simulink model "MMC_idealarm_NLM_SwitchingModel_20251014"  (R2024b)
settings: Solver=FixedStepAuto  StartTime=t_init_sim  StopTime=sim_time  FixedStep=Ts  RelTol=1e-3
InitFcn:
  | param_armsim_20251013
StartFcn:
  | param_armsim_20251013
values from neighbouring files (symbols this model uses):
  a = 1    [param_armsim_20251013.m]
  C_m = 188.4e-6    (= 0.0001884)    [param_armsim_20251013.m]
  f0 = 500    [param_armsim_20251013.m]
  f_control = 10e3    (= 10000)    [param_armsim_20251013.m]
  Fc = 2.5e3    (= 2500)    [param_armsim_20251013.m]
  isAlgoTriActive = true    [param_armsim_20251013.m]
  isPWMActive = false    [param_armsim_20251013.m]
  L_ac = 30e-3    (= 0.03)    [param_armsim_20251013.m]
  m = 1    [param_armsim_20251013.m]
  N = 5    [param_armsim_20251013.m]
  phi = pi/2    (= 1.57079632679)    [param_armsim_20251013.m]
  R_ac = 6    [param_armsim_20251013.m]
  time_charge = 0.2    [param_armsim_20251013.m]
  Ts = 1e-6    (= 1e-06)    [param_armsim_20251013.m]
  VDC = 150    [param_armsim_20251013.m]
undefined symbols (not defined in the file or in its folder): C_SM
libraries: spsVoltageMeasurementLib x8, spsHalfBridgeMMCLib x5, spsSeriesRLCBranchLib x1, spsControlledVoltageSourceLib x1, spsCurrentMeasurementLib x1, spsDiodeLib x1, spsGroundLib x1, spsPWMGeneratorMultilevelLib x1, spspowerguiLib x1
settings Model: Creator=ana  LastModifiedBy=ana

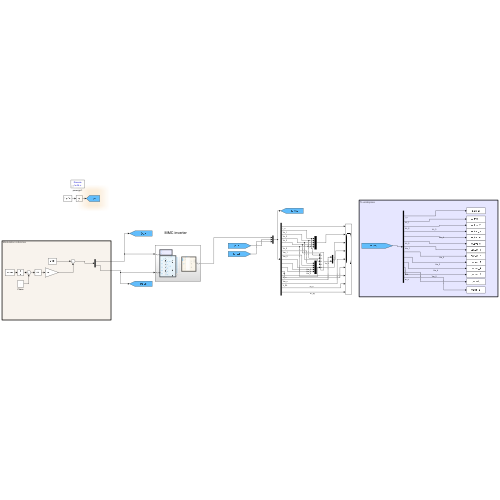
[thumbnail: Simulink's stored preview of the top-level diagram]
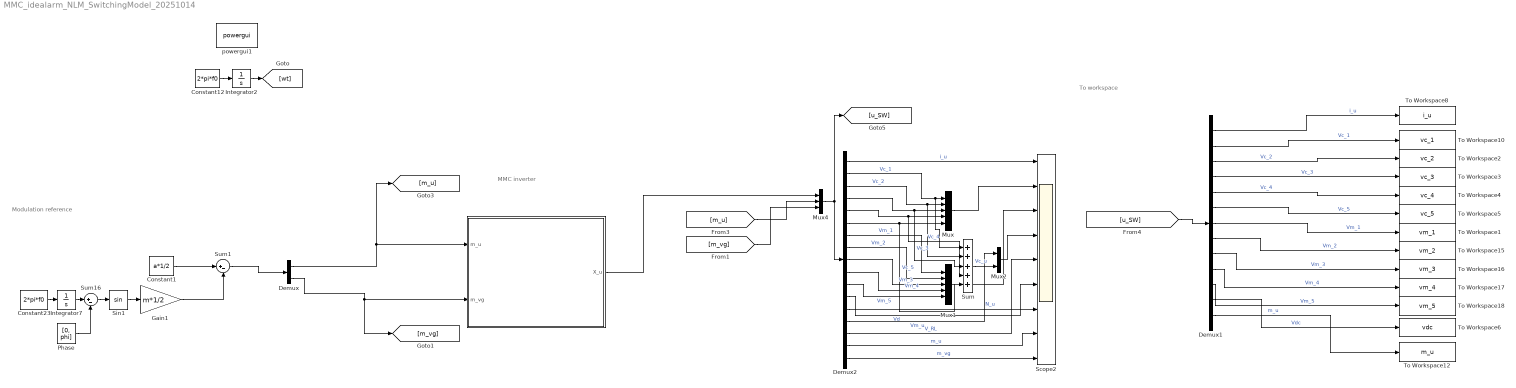
== system MMC_idealarm_NLM_SwitchingModel_20251014 ==
  note: MMC inverter
  note: To workspace
  note: Modulation reference
  " " : Subsystem
  Constant1 : Constant  Value=a*1/2
  Constant12 : Constant  Value=2*pi*f0
  Constant23 : Constant  Value=2*pi*f0
  Demux : Demux  Outputs=2
  Demux1 : Demux  Outputs=13
  Demux2 : Demux  Outputs=17
  Gain1 : Gain  Gain=m*1/2
  Integrator2 : Integrator
  Integrator7 : Integrator
  Mux : Mux  Inputs=5
  Mux1 : Mux  Inputs=5
  Mux2 : Mux  Inputs=2
  Mux4 : Mux  Inputs=3
  Phase : Constant  Value=[0, phi]
  Scope2 : Scope  NumInputPorts=9
  Sin1 : Trigonometry
  Sum : Sum  Inputs=+++++
  Sum1 : Sum  Inputs=|+-
  Sum16 : Sum  Inputs=|+-
  To Workspace1 : ToWorkspace  VariableName=vm_1  SaveFormat=Structure With Time  SampleTime=-1
      settings: MaxDataPoints=10*200000
  To Workspace10 : ToWorkspace  VariableName=vc_1  SaveFormat=Structure With Time  SampleTime=-1
      settings: MaxDataPoints=10*200000
  To Workspace12 : ToWorkspace  VariableName=m_u  SaveFormat=Structure With Time  SampleTime=-1
      settings: MaxDataPoints=10*200000
  To Workspace15 : ToWorkspace  VariableName=vm_2  SaveFormat=Structure With Time  SampleTime=-1
      settings: MaxDataPoints=10*200000
  To Workspace16 : ToWorkspace  VariableName=vm_3  SaveFormat=Structure With Time  SampleTime=-1
      settings: MaxDataPoints=10*200000
  To Workspace17 : ToWorkspace  VariableName=vm_4  SaveFormat=Structure With Time  SampleTime=-1
      settings: MaxDataPoints=10*200000
  To Workspace18 : ToWorkspace  VariableName=vm_5  SaveFormat=Structure With Time  SampleTime=-1
      settings: MaxDataPoints=10*200000
  To Workspace2 : ToWorkspace  VariableName=vc_2  SaveFormat=Structure With Time  SampleTime=-1
      settings: MaxDataPoints=10*200000
  To Workspace3 : ToWorkspace  VariableName=vc_3  SaveFormat=Structure With Time  SampleTime=-1
      settings: MaxDataPoints=10*200000
  To Workspace4 : ToWorkspace  VariableName=vc_4  SaveFormat=Structure With Time  SampleTime=-1
      settings: MaxDataPoints=10*200000
  To Workspace5 : ToWorkspace  VariableName=vc_5  SaveFormat=Structure With Time  SampleTime=-1
      settings: MaxDataPoints=10*200000
  To Workspace6 : ToWorkspace  VariableName=vdc  SaveFormat=Structure With Time  SampleTime=-1
      settings: MaxDataPoints=10*200000
  To Workspace8 : ToWorkspace  VariableName=i_u  SaveFormat=Structure With Time  SampleTime=-1
      settings: MaxDataPoints=10*200000
  powergui1 : spspowerguiLib/powergui  Priority=1  SimulationMode=Discrete  SampleTime=Ts  frequency=60  Iterations=50  frequencyindice=0  Pbase=100e6  ErrMax=1e-4  UnitsV=V  UnitsW=W  buscounter=0  FunctionMessages=off  echomessages=off  EnableUseOfTLC=off  CurrentSourceSwitches=off  DisableSnubberDevices=off  DisableRonSwitches=off  DisableVfSwitches=off  DisplayEquations=off  AutomaticDiscreteSolvers=off  SolverType=Backward Euler  Interpol=off  ExternalGateDelay=off  methode=off  Ts=0  x0status=blocks  SPID=off  SwTol=0  HookPort=off  NonlinearTolerance=1e-4  nMaxIteration=100  ContinueOnMaxIteration=off  RestoreLinks=warning  ResistiveCurrentMeasurement=off  Frange=[0:2:500]  Ylog=off  Xlog=on  ShowGrid=off  save=off  variable=ZData  structure=0  ZoomFFT=off  StartTime=0.0  cycles=1  DisplayStyle=1  fundamental=60  FreqAxis=off  MaxFrequency=1000  frequencyindicesteady=1  RmsSteady=1  display=off
  wires:
  Demux2/7 -> Mux1/1  "Vm_1"
  Demux2/11 -> Mux1/5  "Vm_5"
  Demux2/9 -> Mux1/3  "Vm_3"
  [u_SW] -> Demux1/1
  Demux1/8 -> To Workspace15/1  "Vm_2"
  Demux1/13 -> To Workspace12/1  "m_u"
  Demux2/10 -> Mux1/4  "Vm_4"
  Demux1/10 -> To Workspace17/1  "Vm_4"
  Demux1/5 -> To Workspace4/1  "Vc_4"
  Demux1/12 -> To Workspace6/1  "Vdc"
  Sin1/1 -> Gain1/1
  " "/1(X_u) -> Mux4/1
  Demux2/1 -> Scope2/1  "i_u"
  Sum16/1 -> Sin1/1
  Constant1/1 -> Sum1/1
  Constant23/1 -> Integrator7/1
  Demux2/16 -> Scope2/8  "m_u"
  Demux1/11 -> To Workspace18/1  "Vm_5"
  [m_u] -> Mux4/2
  Integrator7/1 -> Sum16/1
  Demux2/6 -> Sum/5, Mux/5  "Vc_5"
  Mux4/1 -> [u_SW], Demux2/1
  Constant12/1 -> Integrator2/1
  Integrator2/1 -> [wt]
  Demux1/9 -> To Workspace16/1  "Vm_3"
  Demux1/7 -> To Workspace1/1  "Vm_1"
  Demux1/3 -> To Workspace2/1  "Vc_2"
  Demux1/4 -> To Workspace3/1  "Vc_3"
  Demux1/6 -> To Workspace5/1  "Vc_5"
  Gain1/1 -> Sum1/2
  Phase/1 -> Sum16/2
  Demux1/2 -> To Workspace10/1  "Vc_1"
  Demux2/2 -> Sum/1, Mux/1  "Vc_1"
  Demux1/1 -> To Workspace8/1  "i_u"
  Demux2/5 -> Sum/4, Mux/4  "Vc_4"
  Demux2/3 -> Mux/2, Sum/2  "Vc_2"
  Demux2/4 -> Mux/3, Sum/3  "Vc_3"
  Mux/1 -> Scope2/2
  Demux2/8 -> Mux1/2  "Vm_2"
  Mux1/1 -> Scope2/3
  Demux2/13 -> Scope2/7  "N_u"
  Demux/1 -> [m_u], " "/1(m_u)
  Sum1/1 -> Demux/1
  Demux/2 -> " "/2(m_vg), [m_vg]
  [m_vg] -> Mux4/3
  Demux2/17 -> Scope2/9  "m_vg"
  Demux2/12 -> Scope2/6  "Vd"
  Demux2/15 -> Scope2/5  "V_RL"
  Sum/1 -> Mux2/2  "Vc_u"
  Mux2/1 -> Scope2/4
  Demux2/14 -> Mux2/1  "Vm_u"

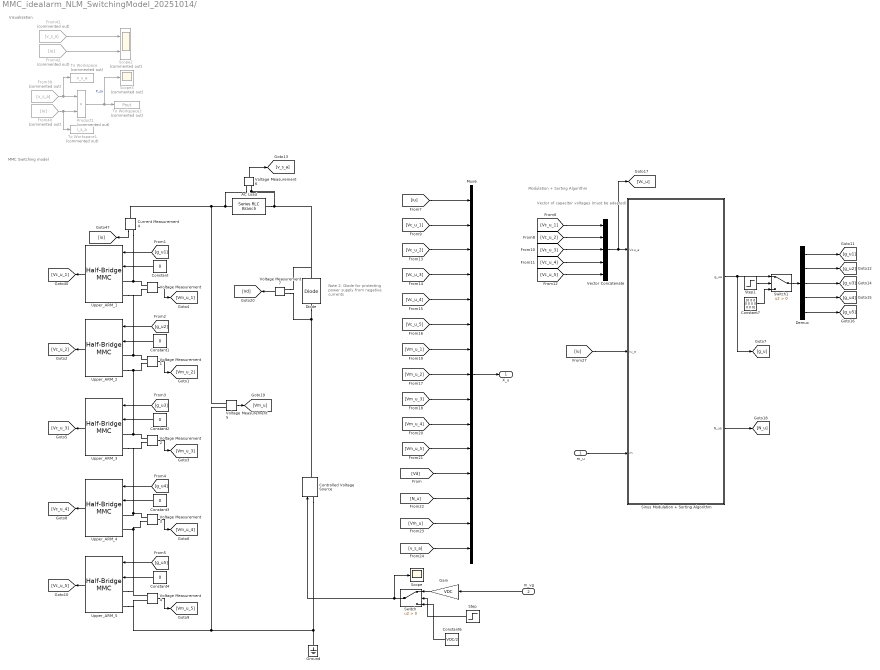
== system MMC_idealarm_NLM_SwitchingModel_20251014/  ==
  note: Vector of capacitor voltages (must be adapted)
  note: Visualisation
  note: Modulation + Sorting Algorithm
  note: MMC Switching model
  note: Note 2:
      | Diode for protecting power supply from negative currents
  m_u : Inport
  m_vg : Inport  Port=2
  AC Load : spsSeriesRLCBranchLib/Series RLC Branch  LConnTagsString=__new0  RConnTagsString=__new0  BranchType=RL  Resistance=R_ac  Inductance=L_ac  SetiL0=off  InitialCurrent=0  Capacitance=C_SM  Setx0=off  InitialVoltage=0  Measurements=None
  Constant{,1..4} (5 alike) : Constant  Value=0
  Constant6 : Constant  Value=VDC/2
  Constant7 : Constant  Value=[0 0 0 0 0 0 0 0 0 0]
  Controlled Voltage Source : spsControlledVoltageSourceLib/Controlled Voltage Source  Initialize=on  Source_Type=AC  Amplitude=VDC/2  Phase=0  Frequency=0  Measurements=None
  Current Measurement4 : spsCurrentMeasurementLib/Current Measurement  PhasorSimulation=off  OutputType=Complex  PSBequivalent=0
  Demux : Demux  Outputs=5
  Diode : spsDiodeLib/Diode  Ron=0.325  Lon=0  Vf=0.4404  IC=0  UseSnubber=0  Rs=1e5  Cs=250e-9  Measurements=off
  From39 : From  Commented=on  GotoTag=v_s_a
  From40 : From  Commented=on  GotoTag=iu
  From41 : From  Commented=on  GotoTag=v_s_a
  From42 : From  Commented=on  GotoTag=iu
  Gain : Gain  Gain=VDC
  Ground : spsGroundLib/Ground  LConnTagsString=a
  Mux6 : Mux  Inputs=15
  Product1 : Product  Commented=on
  Scope : Scope
  Scope2 : Scope  Commented=on  NumInputPorts=2
  Scope3 : Scope  Commented=on
  Sinus Modulation + Sorting Algorithm : Subsystem
  Step : Step  Time=time_charge  SampleTime=0
  Step1 : Step  Time=time_charge  SampleTime=0
  Switch : Switch  Criteria=u2 > Threshold  SaturateOnIntegerOverflow=off  InputSameDT=off
  Switch1 : Switch  Criteria=u2 > Threshold  SaturateOnIntegerOverflow=off  InputSameDT=off
  To Workspace : ToWorkspace  Commented=on  VariableName=v_s_a  SaveFormat=Structure With Time  SampleTime=-1
  To Workspace1 : ToWorkspace  Commented=on  VariableName=i_s_a  SaveFormat=Structure With Time  SampleTime=-1
  To Workspace2 : ToWorkspace  Commented=on  VariableName=Pout  SaveFormat=Structure With Time  SampleTime=-1
  Upper_ARM_{1..5} (5 alike) : spsHalfBridgeMMCLib/Half-Bridge MMC  ModelType=Switching devices  n=1  C=C_m  Vc_Initial=0  Ron=Module_diode_Ron  Rs=Module_snubber_R  Cs=Module_snubber_C  Ron_Diode=1e-3  Rs_Diode=1e6  Cs_Diode=inf  Vf_Diode=1e-3  Rs_CurrentSource=inf  Ts=10e-6
  Vector Concatenate : Concatenate  NumInputs=5
  Voltage Measurement{,1..7} (8 alike) : spsVoltageMeasurementLib/Voltage Measurement  PhasorSimulation=off  OutputType=Complex  PSBequivalent=0
  X_u : Outport
  wires:
  [Vc_u_1] -> Mux6/2
  Mux6/1 -> X_u/1
  Current Measurement4/1 -> [iu]
  Sinus Modulation + Sorting Algorithm/1(g_ua) -> [g_u], Switch1/1
  [iu] -> Sinus Modulation + Sorting Algorithm/2(iu_a)
  Vector Concatenate/1 -> [Vc_u], Sinus Modulation + Sorting Algorithm/1(Vcu_a)
  m_u/1 -> Sinus Modulation + Sorting Algorithm/3(m)
  Product1/1 -> Scope3/1, To Workspace2/1  "P_sa"
  Voltage Measurement6/1 -> [v_s_a]
  From39/1 -> To Workspace/1, Product1/1
  From40/1 -> Product1/2, To Workspace1/1
  From41/1 -> Scope2/1
  From42/1 -> Scope2/2
  Upper_ARM_1/1 -> [Vc_u_1]
  Voltage Measurement/1 -> [Vm_u_1]
  Constant/1 -> Upper_ARM_1/2
  [g_u1] -> Upper_ARM_1/1
  Voltage Measurement1/1 -> [Vm_u_2]
  Upper_ARM_2/1 -> [Vc_u_2]
  Constant1/1 -> Upper_ARM_2/2
  [g_u2] -> Upper_ARM_2/1
  [g_u3] -> Upper_ARM_3/1
  Upper_ARM_3/1 -> [Vc_u_3]
  Constant2/1 -> Upper_ARM_3/2
  Voltage Measurement2/1 -> [Vm_u_3]
  [g_u4] -> Upper_ARM_4/1
  Upper_ARM_4/1 -> [Vc_u_4]
  Constant3/1 -> Upper_ARM_4/2
  Voltage Measurement3/1 -> [Vm_u_4]
  [g_u5] -> Upper_ARM_5/1
  Upper_ARM_5/1 -> [Vc_u_5]
  Constant4/1 -> Upper_ARM_5/2
  Voltage Measurement4/1 -> [Vm_u_5]
  [Vc_u_1] -> Vector Concatenate/1
  [Vc_u_2] -> Vector Concatenate/2
  [Vc_u_3] -> Vector Concatenate/3
  [Vc_u_4] -> Vector Concatenate/4
  [Vc_u_5] -> Vector Concatenate/5
  Demux/1 -> [g_u1]
  Demux/2 -> [g_u2]
  Demux/3 -> [g_u3]
  Demux/4 -> [g_u4]
  Demux/5 -> [g_u5]
  [iu] -> Mux6/1
  [Vc_u_2] -> Mux6/3
  [Vc_u_3] -> Mux6/4
  [Vc_u_4] -> Mux6/5
  [Vc_u_5] -> Mux6/6
  [Vm_u_1] -> Mux6/7
  [Vm_u_2] -> Mux6/8
  [Vm_u_3] -> Mux6/9
  [Vm_u_4] -> Mux6/10
  [Vm_u_5] -> Mux6/11
  [Vd] -> Mux6/12
  m_vg/1 -> Gain/1
  Sinus Modulation + Sorting Algorithm/2(N_ua) -> [N_u]
  [N_u] -> Mux6/13
  Voltage Measurement5/1 -> [Vm_u]
  [Vm_u] -> Mux6/14
  [v_s_a] -> Mux6/15
  Gain/1 -> Switch/1
  Switch/1 -> Scope/1, Controlled Voltage Source/1
  Constant6/1 -> Switch/3
  Switch1/1 -> Demux/1
  Constant7/1 -> Switch1/3
  Step/1 -> Switch/2
  Step1/1 -> Switch1/2
  Voltage Measurement7/1 -> [Vd]
  connections:
  Voltage Measurement4/LConn2 -- Upper_ARM_5/LConn2 -- Voltage Measurement5/LConn2 -- Controlled Voltage Source/LConn1 -- Ground/LConn1
  Voltage Measurement/LConn1 -- Current Measurement4/RConn1 -- Upper_ARM_1/LConn1
  Voltage Measurement6/LConn1 -- Voltage Measurement7/LConn1 -- Diode/RConn1 -- AC Load/LConn1
  Voltage Measurement6/LConn2 -- AC Load/RConn1 -- Voltage Measurement5/LConn1 -- Current Measurement4/LConn1
  Voltage Measurement1/LConn1 -- Voltage Measurement/LConn2 -- Upper_ARM_1/LConn2 -- Upper_ARM_2/LConn1
  Voltage Measurement1/LConn2 -- Upper_ARM_2/LConn2 -- Voltage Measurement2/LConn1 -- Upper_ARM_3/LConn1
  Voltage Measurement3/LConn2 -- Voltage Measurement4/LConn1 -- Upper_ARM_5/LConn1 -- Upper_ARM_4/LConn2
  Voltage Measurement3/LConn1 -- Voltage Measurement2/LConn2 -- Upper_ARM_3/LConn2 -- Upper_ARM_4/LConn1
  Diode/LConn1 -- Voltage Measurement7/LConn2 -- Controlled Voltage Source/RConn1

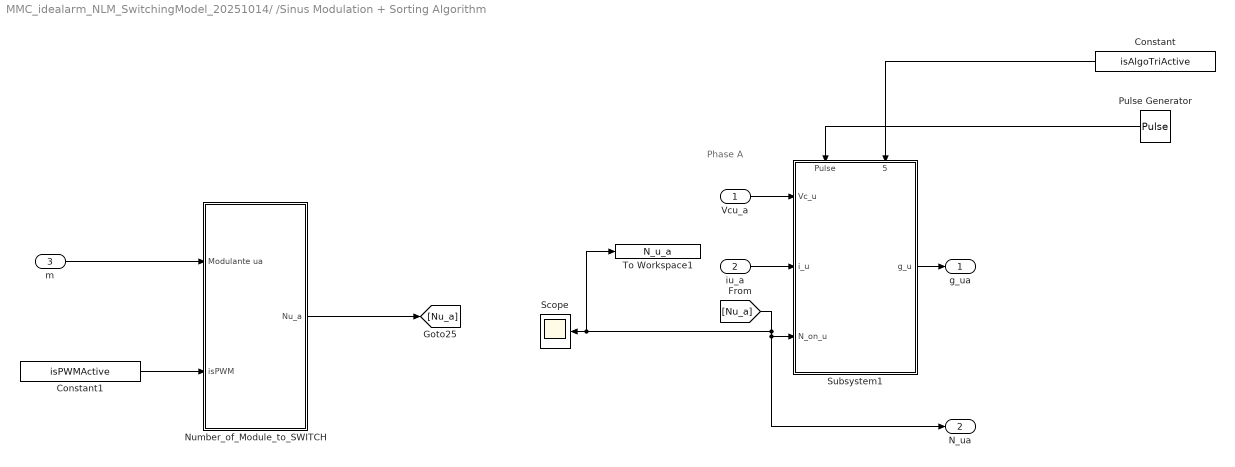
== system MMC_idealarm_NLM_SwitchingModel_20251014/ /Sinus Modulation + Sorting Algorithm ==
  note: Phase A
  Vcu_a : Inport
  iu_a : Inport  Port=2
  m : Inport  Port=3
  Constant : Constant  Value=isAlgoTriActive
  Constant1 : Constant  Value=isPWMActive
  Number_of_Module_to_SWITCH : Subsystem
  Pulse Generator : DiscretePulseGenerator  PulseType=Time based  Period=1/f_control  PulseWidth=5  SampleTime=1/(N*Fc)
  Scope : Scope
  Subsystem1 : Subsystem
      settings: PortSchema="{\"entries\":[{\"content\":{\"sides\":[{\"content\":{\"connectorIds\":[\"In1\",\"In2\",\"In3\"]},\"type\":\"ConnectorPlacement.EquallySpacedRectSide\",\"uuid\":\"edb50160-a239-40a6-972c-a715a6fbe13d\"},{\"content\":{\"connectorIds\":[\"Out1\"],\"side\":\"RIGHT\"},\"type\":\"ConnectorPlacement.EquallySpacedRectSide\",\"uuid\":\"50795e67-0526-4c95-8fde-c2f33aa10269\"},{\"content\":{\"connectorIds\":[\"In4\",\"In5\"],\"side\":\"TOP\"},\"type\":\"ConnectorPlacement.EquallySpacedRectSide\",\"uuid\":\"4b9fa748-0c00-40fa-8ad9-db170ea8506d\"}]},\"type\":\"ConnectorPlacement.EquallySpacedConnector\",\"uuid\":\"80f12ca1-3964-4a1c-b648-ca12c0c72645\"}],\"packageUris\":[\"http://schema.mathworks.com/mf0/Connector/R2020b\"],\"version\":\"1.0\"}"
  To Workspace1 : ToWorkspace  VariableName=N_u_a  SaveFormat=Structure With Time  SampleTime=-1
  g_ua : Outport
  N_ua : Outport  Port=2
  wires:
  Vcu_a/1 -> Subsystem1/1(Vc_u)
  iu_a/1 -> Subsystem1/2(i_u)
  [Nu_a] -> N_ua/1, Subsystem1/3(N_on_u), To Workspace1/1, Scope/1
  Number_of_Module_to_SWITCH/1(Nu_a) -> [Nu_a]
  Subsystem1/1(g_u) -> g_ua/1
  Pulse Generator/1 -> Subsystem1/4(Pulse)
  m/1 -> Number_of_Module_to_SWITCH/1(Modulante ua)
  Constant/1 -> Subsystem1/5(isAlgoTriActive)
  Constant1/1 -> Number_of_Module_to_SWITCH/2(isPWM)

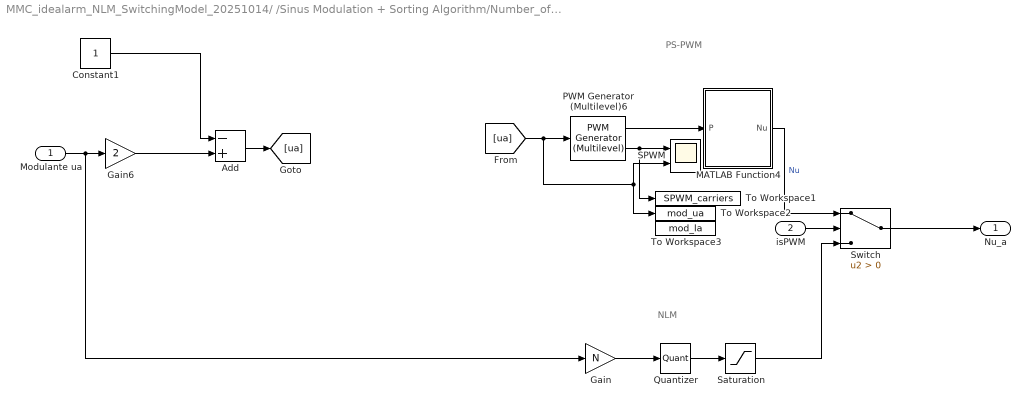
== system MMC_idealarm_NLM_SwitchingModel_20251014/ /Sinus Modulation + Sorting Algorithm/Number_of_Module_to_SWITCH ==
  note: PS-PWM
  note: NLM
  Modulante ua : Inport
  isPWM : Inport  Port=2
  Add : Sum  Inputs=-+
  Constant1 : Constant
  Gain : Gain  Gain=N
  Gain6 : Gain  Gain=2
  MATLAB Function4 : MATLAB Function  TreatAsAtomicUnit=on
  PWM Generator (Multilevel)6 : spsPWMGeneratorMultilevelLib/PWM Generator (Multilevel)  BridgeType=Half-bridge  NumberOfBridges=N  Fc=Fc  Ts=0  ShowCarriersOutport=on
  Quantizer : Quantizer  QuantizationInterval=1
  SPWM : Scope  NumInputPorts=2
  Saturation : Saturate  UpperLimit=5  LowerLimit=0
  Switch : Switch  Criteria=u2 > Threshold  SaturateOnIntegerOverflow=off  InputSameDT=off
  To Workspace1 : ToWorkspace  VariableName=SPWM_carriers  SaveFormat=Structure With Time  SampleTime=-1
  To Workspace2 : ToWorkspace  VariableName=mod_ua  SaveFormat=Structure With Time  SampleTime=-1
  To Workspace3 : ToWorkspace  VariableName=mod_la  SaveFormat=Structure With Time  SampleTime=-1
  Nu_a : Outport
  wires:
  Modulante ua/1 -> Gain/1, Gain6/1
  PWM Generator (Multilevel)6/1 -> MATLAB Function4/1(P)
  [ua] -> To Workspace2/1, SPWM/2, PWM Generator (Multilevel)6/1
  MATLAB Function4/1(Nu) -> Switch/1  "Nu"
  Gain6/1 -> Add/2
  Add/1 -> [ua]
  Constant1/1 -> Add/1
  PWM Generator (Multilevel)6/2 -> To Workspace1/1, SPWM/1
  Gain/1 -> Quantizer/1
  Quantizer/1 -> Saturation/1
  Saturation/1 -> Switch/3
  isPWM/1 -> Switch/2
  Switch/1 -> Nu_a/1

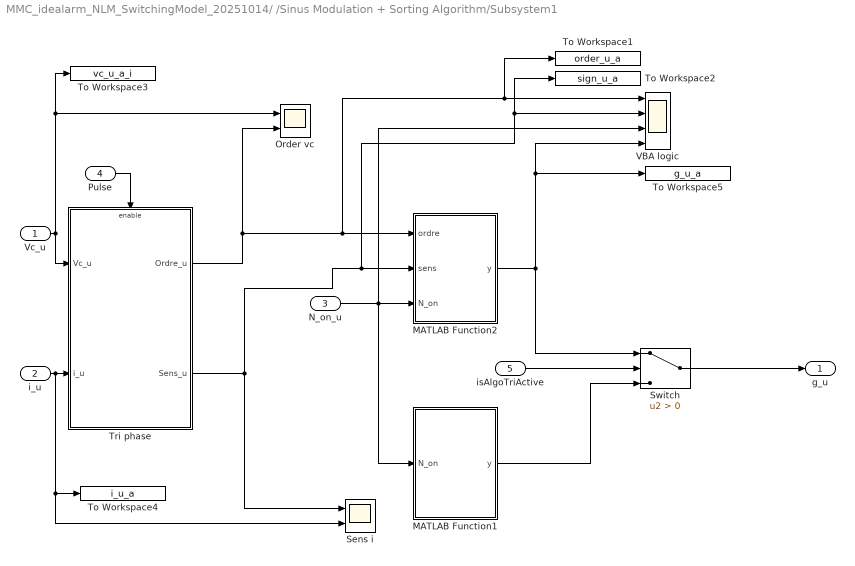
== system MMC_idealarm_NLM_SwitchingModel_20251014/ /Sinus Modulation + Sorting Algorithm/Subsystem1 ==
  Vc_u : Inport
  i_u : Inport  Port=2
  N_on_u : Inport  Port=3
  Pulse : Inport  Port=4
  isAlgoTriActive : Inport  Port=5
  MATLAB Function1 : MATLAB Function  TreatAsAtomicUnit=on
  MATLAB Function2 : MATLAB Function  TreatAsAtomicUnit=on
  Order vc : Scope  NumInputPorts=2
  Sens i : Scope  NumInputPorts=2
  Switch : Switch  Criteria=u2 > Threshold  SaturateOnIntegerOverflow=off  InputSameDT=off
  To Workspace1 : ToWorkspace  VariableName=order_u_a  SaveFormat=Structure With Time  SampleTime=-1
  To Workspace2 : ToWorkspace  VariableName=sign_u_a  SaveFormat=Structure With Time  SampleTime=-1
  To Workspace3 : ToWorkspace  VariableName=vc_u_a_i  SaveFormat=Structure With Time  SampleTime=-1
  To Workspace4 : ToWorkspace  VariableName=i_u_a  SaveFormat=Structure With Time  SampleTime=-1
  To Workspace5 : ToWorkspace  VariableName=g_u_a  SaveFormat=Structure With Time  SampleTime=-1
  Tri phase : Subsystem
  VBA logic : Scope  NumInputPorts=4
  g_u : Outport
  wires:
  Vc_u/1 -> To Workspace3/1, Order vc/1, Tri phase/1(Vc_u)
  Tri phase/1(Ordre_u) -> To Workspace1/1, VBA logic/1, MATLAB Function2/1(ordre), Order vc/2
  N_on_u/1 -> MATLAB Function1/1(N_on), VBA logic/3, MATLAB Function2/3(N_on)
  i_u/1 -> To Workspace4/1, Sens i/2, Tri phase/2(i_u)
  Tri phase/2(Sens_u) -> VBA logic/2, To Workspace2/1, MATLAB Function2/2(sens), Sens i/1
  Pulse/1 -> Tri phase/Enable
  MATLAB Function2/1(y) -> Switch/1, To Workspace5/1, VBA logic/4
  isAlgoTriActive/1 -> Switch/2
  MATLAB Function1/1(y) -> Switch/3
  Switch/1 -> g_u/1

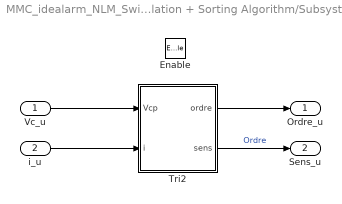
== system MMC_idealarm_NLM_SwitchingModel_20251014/ /Sinus Modulation + Sorting Algorithm/Subsystem1/Tri phase ==
  Vc_u : Inport
  i_u : Inport  Port=2
  Enable : EnablePort
  Tri2 : MATLAB Function  TreatAsAtomicUnit=on
  Ordre_u : Outport
  Sens_u : Outport  Port=2
  wires:
  Vc_u/1 -> Tri2/1(Vcp)
  i_u/1 -> Tri2/2(i)
  Tri2/1(ordre) -> Ordre_u/1
  Tri2/2(sens) -> Sens_u/1  "Ordre"

== matlab function MMC_idealarm_NLM_SwitchingModel_20251014/ /Sinus Modulation + Sorting Algorithm/Subsystem1/MATLAB Function1 ==
  data: y output; N_on input
function y = fcn(N_on)
ordre = [1 2 3 4 5];
sens = 1;
N_m = length(ordre);
Gp = zeros(1,2*N_m);
Ap0=ordre;

%% Sens positif (sens = 1)
if sens==1         % ON les condensateurs les moins chargés
    
    %K1 = 1 ; K2 = 0
    kp = 1:N_on;
    Gp(2*Ap0(kp))=0;
    Gp(2*Ap0(kp)-1)=1;
    
    %K1 = 0 ; K2 = 1
    kp = N_on+1:N_m;
    Gp(2*Ap0(kp))=1;
    Gp(2*Ap0(kp)-1)=0;

else            % ON les condensateurs les plus chargés
    
    %K1 = 1 ; K2 = 0
    kp = N_m:-1:N_m+1-N_on;
    Gp(2*Ap0(kp))=0;
    Gp(2*Ap0(kp)-1)=1;
    
    %K1 = 0 ; K2 = 1
    kp = N_m-N_on:-1:1;
    Gp(2*Ap0(kp))=1;
    Gp(2*Ap0(kp)-1)=0;
end
y=Gp;

== matlab function MMC_idealarm_NLM_SwitchingModel_20251014/ /Sinus Modulation + Sorting Algorithm/Number_of_Module_to_SWITCH/MATLAB Function4 ==
  data: Nu output; P input
function Nu = fcn(P)

s=0;

for k = 1:2:length(P)
    s=s+P(k);
end

Nu=s;

== matlab function MMC_idealarm_NLM_SwitchingModel_20251014/ /Sinus Modulation + Sorting Algorithm/Subsystem1/Tri phase/Tri2 ==
  data: ordre output; Vcp input; i input; sens output
function [ordre,sens] = fcn(Vcp, i)

[~, ordre] = sort(Vcp);

if i > 0 
    sens = 1;
else 
    sens = 0;
end

== matlab function MMC_idealarm_NLM_SwitchingModel_20251014/ /Sinus Modulation + Sorting Algorithm/Subsystem1/MATLAB Function2 ==
  data: ordre input; y output; sens input; N_on input
function y = fcn(ordre,sens,N_on)

N_m = length(ordre);
Gp = zeros(1,2*N_m);
Ap0=ordre;

%% Sens positif (sens = 1)
if sens==1         % ON les condensateurs les moins chargés
    
    %K1 = 1 ; K2 = 0
    kp = 1:N_on;
    Gp(2*Ap0(kp))=0;
    Gp(2*Ap0(kp)-1)=1;
    
    %K1 = 0 ; K2 = 1
    kp = N_on+1:N_m;
    Gp(2*Ap0(kp))=1;
    Gp(2*Ap0(kp)-1)=0;

else            % ON les condensateurs les plus chargés
    
    %K1 = 1 ; K2 = 0
    kp = N_m:-1:N_m+1-N_on;
    Gp(2*Ap0(kp))=0;
    Gp(2*Ap0(kp)-1)=1;
    
    %K1 = 0 ; K2 = 1
    kp = N_m-N_on:-1:1;
    Gp(2*Ap0(kp))=1;
    Gp(2*Ap0(kp)-1)=0;
end
y=Gp;
